simulink model "R7014E_QuadTankSim"  (R2024a)
settings: Solver=ode4  StartTime=0.0  StopTime=inf  FixedStep=0.01  RelTol=1e-3  EnableMultiTasking=on
values from neighbouring files (symbols this model uses):
  d2 = 0.057 * 0.25    (= 0.01425)    [IMC.m]
  denG11 = denG11{1}    [IMC.m]
  denG22 = denG22{1}    [IMC.m]
  denQ1 = denQ1{1}    [IMC.m]
  denQ2 = denQ2{1}    [IMC.m]
  numG11 = numG11{1}    [IMC.m]
  numG22 = numG22{1}    [IMC.m]
  numQ1 = numQ1{1}    [IMC.m]
  numQ2 = numQ2{1}    [IMC.m]
undefined symbols (not defined in the file or in its folder): linear_params
Description:
  | Double tank process simulation model
  | V1.0
  | 
  | Author: Wolfgang Birk, LTU
settings Model: MinMaxOverflowLogging=ForceOff  PacingRate=18  Creator=wolfgang  LastModifiedBy=geopap-4
settings SolverCC: AlgebraicLoopSolver=TrustRegion
settings DataIOCC: LimitDataPoints=on  SaveFormat=Array  SignalLoggingSaveFormat=ModelDataLogs  ReturnWorkspaceOutputs=off
settings OptimizationCC: ExpressionDepthLimit=2147483647  LifeSpan=inf
settings DebuggingCC: UnderspecifiedInitializationDetection=Classic  MergeDetectMultiDrivingBlocksExec=none  SolverPrmCheckMsg=warning  FcnCallInpInsideContextMsg=warning  UnconnectedInputMsg=warning  UnconnectedOutputMsg=warning  UnconnectedLineMsg=warning  StateNameClashWarn=warning  SFUnexpectedBacktrackingDiag=warning  SFNoUnconditionalDefaultTransitionDiag=warning  SFExecutionAtInitializationDiag=none  ArithmeticOperatorsInVariantConditions=warning
settings HardwareCC: ProdBitPerPointer=32  ProdBitPerSizeT=32  ProdBitPerPtrDiffT=32  ProdLargestAtomicFloat=None  ProdIntDivRoundTo=Undefined  ProdEndianess=Unspecified  ProdWordSize=32  ProdHWDeviceType=32-bit Generic
settings ModelReferenceCC: EnableRefExpFcnMdlSchedulingChecks=on  PropagateSignalLabelsOutOfModel=off
settings SFSimCC: SimUseLocalCustomCode=off  CustomCodeUndefinedFunction=UseInterfaceOnly
settings RTWCC: RTWUseLocalCustomCode=off  GPUComputeCapability=3.5
settings CodeAppCC: StateflowObjectComments=on
settings GRTTargetCC: TargetLangStandard=C89/C90 (ANSI)
settings ConfigComp: CovMetricSettings=dw  CovSaveCumulativeToWorkspaceVar=on  CovSaveSingleToWorkspaceVar=on  CovExternalEMLEnable=off

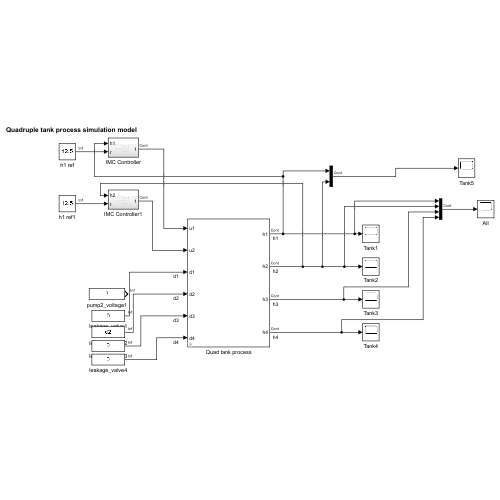
[thumbnail: Simulink's stored preview of the top-level diagram]
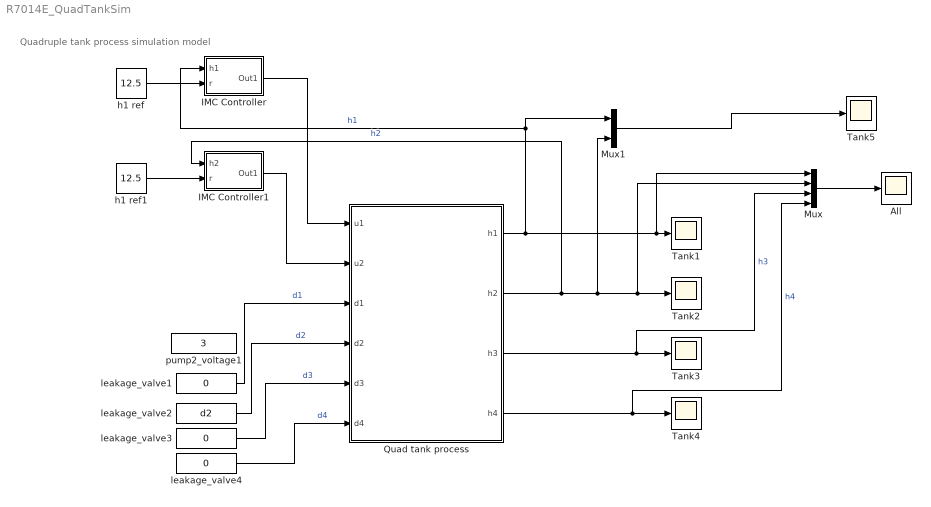
== system R7014E_QuadTankSim ==
  note: Quadruple tank process simulation model
  All : Scope
  IMC Controller : Subsystem
  IMC Controller1 : Subsystem
  Mux : Mux
  Mux1 : Mux  Inputs=2
  Quad tank process : Subsystem  mask{hmax=linear_params.tank_height, A1=linear_params.tank1_area, ao1=linear_params.tank1_opening, h10=linear_params.initial_level1, A2=linear_params.tank2_area, ao2=linear_params.tank2_opening, h20=linear_params.initial_level2, A3=linear_params.tank3_area, ao3=linear_params.tank3_opening, h30=linear_params.initial_level3, A4=linear_params.tank4_area, ao4=linear_params.tank4_opening, h40=linear_params.initial_level4, k1=linear_params.pump1_gain, k2=linear_params.pump2_gain, gamma1=linear_params.split_valve_gamma1, gamma2=linear_params.split_valve_gamma2}
      mask prompts: hmax "Tank height (cm)"; A1 "Tank area (cm^2)"; ao1 "Opening area (cm^2)"; h10 "Initial level (cm)"; A2 "Tank area (cm^2)"; ao2 "Opening area (cm^2)"; h20 "Initial level (cm)"; A3 "Tank area (cm^2)"; ao3 "Opening area (cm^2)"; h30 "Initial level (cm)"; A4 "Tank area (cm^2)"; ao4 "Opening area (cm^2)"; h40 "Initial level (cm)"; k1 "Pump1 gain (cm^3/V/s)"; k2 "Pump2 gain (cm^3/V/s)"; gamma1 "Split valve gamma 1"; gamma2 "Split valve gamma 2"
      mask help: Double tank process parameters
      mask DialogControl Container3 Prompt: General parameters
      mask DialogControl ParameterGroupVar Prompt: Tank 1
      mask DialogControl ParameterGroupVar_copy_copy_copy Prompt: Tank 2
      mask DialogControl ParameterGroupVar_copy_copy Prompt: Tank 3
      mask DialogControl ParameterGroupVar_copy Prompt: Tank 4
      mask DialogControl Container4 Prompt: Pump parameters
  Tank{1..5} (5 alike) : Scope
  h1 ref : Constant  Value=12.5
  h1 ref1 : Constant  Value=12.5
  leakage_valve1 : Constant  Value=0
  leakage_valve2 : Constant  Value=d2
  leakage_valve3 : Constant  Value=0
  leakage_valve4 : Constant  Value=0
  pump2_voltage1 : Constant  Value=3
  wires:
  Quad tank process/3(h3) -> Mux/3, Tank3/1  "h3"
  Quad tank process/1(h1) -> Mux/1, Tank1/1, Mux1/1, IMC Controller/1(h1)  "h1"
  leakage_valve1/1 -> Quad tank process/3(d1)  "d1"
  leakage_valve2/1 -> Quad tank process/4(d2)  "d2"
  leakage_valve3/1 -> Quad tank process/5(d3)  "d3"
  leakage_valve4/1 -> Quad tank process/6(d4)  "d4"
  Quad tank process/2(h2) -> IMC Controller1/1(h2), Mux1/2, Mux/2, Tank2/1  "h2"
  Quad tank process/4(h4) -> Mux/4, Tank4/1  "h4"
  Mux/1 -> All/1
  IMC Controller/1(Out1) -> Quad tank process/1(u1)
  h1 ref/1 -> IMC Controller/2(r)
  IMC Controller1/1(Out1) -> Quad tank process/2(u2)
  h1 ref1/1 -> IMC Controller1/2(r)
  Mux1/1 -> Tank5/1

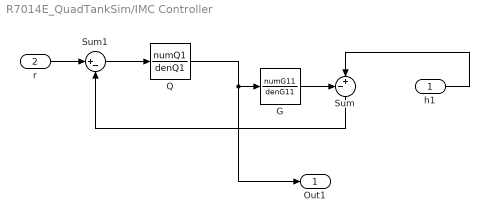
== system R7014E_QuadTankSim/IMC Controller ==
  h1 : Inport
  r : Inport  Port=2
  G : TransferFcn  Numerator=numG11  Denominator=denG11
  Q : TransferFcn  Numerator=numQ1  Denominator=denQ1
  Sum : Sum  Inputs=-+|
  Sum1 : Sum  Inputs=|+-
  Out1 : Outport
  wires:
  Sum1/1 -> Q/1
  Sum/1 -> Sum1/2
  G/1 -> Sum/1
  h1/1 -> Sum/2
  Q/1 -> Out1/1, G/1
  r/1 -> Sum1/1

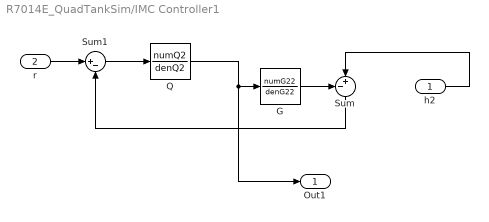
== system R7014E_QuadTankSim/IMC Controller1 ==
  h2 : Inport
  r : Inport  Port=2
  G : TransferFcn  Numerator=numG22  Denominator=denG22
  Q : TransferFcn  Numerator=numQ2  Denominator=denQ2
  Sum : Sum  Inputs=-+|
  Sum1 : Sum  Inputs=|+-
  Out1 : Outport
  wires:
  Sum1/1 -> Q/1
  Sum/1 -> Sum1/2
  G/1 -> Sum/1
  h2/1 -> Sum/2
  Q/1 -> Out1/1, G/1
  r/1 -> Sum1/1

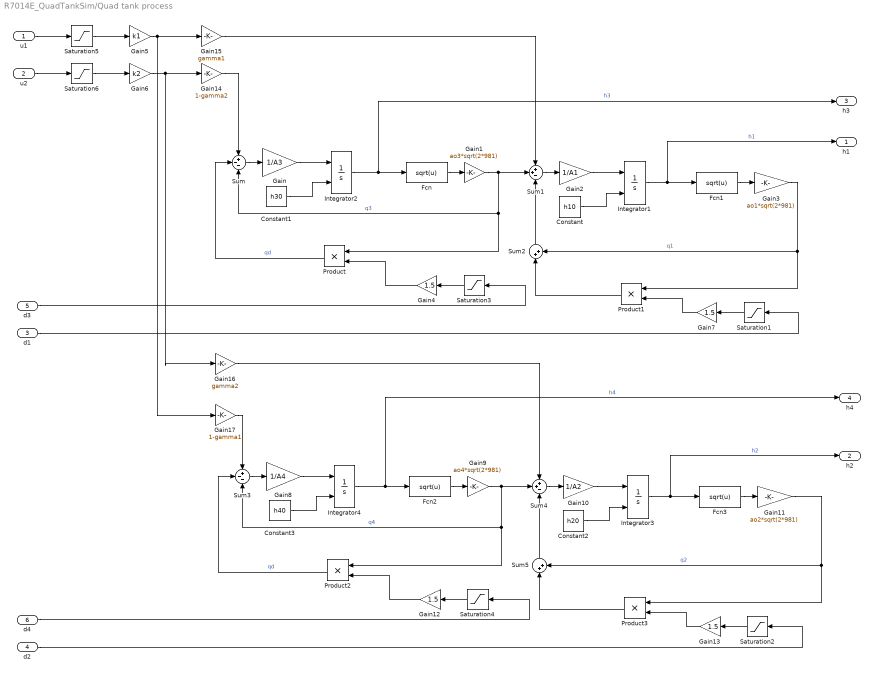
== system R7014E_QuadTankSim/Quad tank process ==
  u1 : Inport
  u2 : Inport  Port=2
  d1 : Inport  Port=3
  d2 : Inport  Port=4
  d3 : Inport  Port=5
  d4 : Inport  Port=6
  Constant : Constant  Value=h10
  Constant1 : Constant  Value=h30
  Constant2 : Constant  Value=h20
  Constant3 : Constant  Value=h40
  Fcn{,1..3} (4 alike) : Fcn  Expr=sqrt(u)
  Gain : Gain  Gain=1/A3
  Gain1 : Gain  Gain=ao3*sqrt(2*981)
  Gain10 : Gain  Gain=1/A2
  Gain11 : Gain  Gain=ao2*sqrt(2*981)
  Gain{4,7,12..13} (4 alike) : Gain  Gain=1.5
  Gain14 : Gain  Gain=1-gamma2
  Gain15 : Gain  Gain=gamma1
  Gain16 : Gain  Gain=gamma2
  Gain17 : Gain  Gain=1-gamma1
  Gain2 : Gain  Gain=1/A1
  Gain3 : Gain  Gain=ao1*sqrt(2*981)
  Gain5 : Gain  Gain=k1
  Gain6 : Gain  Gain=k2
  Gain8 : Gain  Gain=1/A4
  Gain9 : Gain  Gain=ao4*sqrt(2*981)
  Integrator{1..4} (4 alike) : Integrator  InitialConditionSource=external  LimitOutput=on  UpperSaturationLimit=hmax  LowerSaturationLimit=0
  Product{,1..3} (4 alike) : Product  RndMeth=Zero
  Saturation{1..4} (4 alike) : Saturate  UpperLimit=1  LowerLimit=0
  Saturation5 : Saturate  UpperLimit=10  LowerLimit=0
  Saturation6 : Saturate  UpperLimit=10  LowerLimit=0
  Sum : Sum  Inputs=+--
  Sum1 : Sum  Inputs=++-
  Sum2 : Sum  Inputs=|++
  Sum3 : Sum  Inputs=+--
  Sum4 : Sum  Inputs=++-
  Sum5 : Sum  Inputs=|++
  h1 : Outport  VectorParamsAs1DForOutWhenUnconnected=off
  h2 : Outport  Port=2  VectorParamsAs1DForOutWhenUnconnected=off
  h3 : Outport  Port=3  VectorParamsAs1DForOutWhenUnconnected=off
  h4 : Outport  Port=4  VectorParamsAs1DForOutWhenUnconnected=off
  wires:
  Sum/1 -> Gain/1
  Gain/1 -> Integrator2/1
  Fcn/1 -> Gain1/1
  Gain1/1 -> Product/1, Sum/3, Sum1/2  "q3"
  Sum1/1 -> Gain2/1
  Gain2/1 -> Integrator1/1
  Fcn1/1 -> Gain3/1
  Integrator2/1 -> h3/1, Fcn/1  "h3"
  Product/1 -> Sum/2  "qd"
  d3/1 -> Saturation3/1
  Integrator1/1 -> h1/1, Fcn1/1  "h1"
  Saturation3/1 -> Gain4/1
  Gain4/1 -> Product/2
  u1/1 -> Saturation5/1
  Constant/1 -> Integrator1/2
  Constant1/1 -> Integrator2/2
  u2/1 -> Saturation6/1
  Gain5/1 -> Gain17/1, Gain15/1
  Sum2/1 -> Sum1/3
  Gain3/1 -> Product1/1, Sum2/2  "q1"
  Gain7/1 -> Product1/2
  Saturation1/1 -> Gain7/1
  d1/1 -> Saturation1/1
  Product1/1 -> Sum2/1
  Product3/1 -> Sum5/1
  d2/1 -> Saturation2/1
  Saturation2/1 -> Gain13/1
  Gain13/1 -> Product3/2
  Gain11/1 -> Sum5/2, Product3/1  "q2"
  Sum5/1 -> Sum4/3
  Constant3/1 -> Integrator4/2
  Constant2/1 -> Integrator3/2
  Gain12/1 -> Product2/2
  Saturation4/1 -> Gain12/1
  Integrator3/1 -> Fcn3/1, h2/1  "h2"
  d4/1 -> Saturation4/1
  Product2/1 -> Sum3/2  "qd"
  Integrator4/1 -> h4/1, Fcn2/1  "h4"
  Fcn3/1 -> Gain11/1
  Gain10/1 -> Integrator3/1
  Sum4/1 -> Gain10/1
  Gain9/1 -> Sum4/2, Sum3/3, Product2/1  "q4"
  Fcn2/1 -> Gain9/1
  Gain8/1 -> Integrator4/1
  Sum3/1 -> Gain8/1
  Gain14/1 -> Sum/1
  Gain15/1 -> Sum1/1
  Gain6/1 -> Gain16/1, Gain14/1
  Gain16/1 -> Sum4/1
  Gain17/1 -> Sum3/1
  Saturation5/1 -> Gain5/1
  Saturation6/1 -> Gain6/1
